simulink model "Demo_PreScanCarSim3D_cs"  (Simulink 7.6)
settings: Solver=ode5  SolverMode=SingleTasking  StartTime=0.0  StopTime=68  FixedStep=1/400  RelTol=1e-3
PreLoadFcn:
  | check_NUTS_defined;
  | 
  | assignin('base',['model_closed_' bdroot],false);
InitFcn:
  | PreScanExperimentInitFcn(bdroot)
StopFcn:
  | PreScanExperimentStopFcn(bdroot)
undefined symbols (not defined in the file or in its folder): DiscIntNeverNeededParam, warningInitialVelocity, x0, x_ini_VRML, y_ini_VRML, z_ini_VRML
libraries: PreScanSimulinkLibrary x13, simulink_extras x5, PreScanUsefulBlocks x5, simulink x3, Solver_SF x1
(part 6 of 10)

== system Demo_PreScanCarSim3D_cs/VISUCasingLights_TrafficLightRoadSideNL_2/conv_Green ==
  on_off : Inport
  Constant5 : Constant  Value=[5 32 25 255 0 64 50 255 0 64 50 255 0 0 0 255]
  Constant9 : Constant  Value="[0 45 34 255  0 45 34 255  0 45 34 255  30 306 240 255]"
  Switch2 : Switch  Threshold=0.5
  RGBcolor : Outport
  wires:
  Switch2/1 -> RGBcolor/1
  on_off/1 -> Switch2/2
  Constant5/1 -> Switch2/3  "off"
  Constant9/1 -> Switch2/1  "on"

== system Demo_PreScanCarSim3D_cs/VISUCasingLights_TrafficLightRoadSideNL_2/conv_Orange ==
  on_off : Inport
  Constant2 : Constant  Value="[45 34 0 255  45 34 0 255  45 34 0 255  306 229 5 255]"
  Constant20 : Constant  Value=[32 25 5 255 64 48 5 255 64 54 5 255 0 0 0 255]
  Switch1 : Switch  Threshold=0.5
  RGBcolor : Outport
  wires:
  Constant20/1 -> Switch1/3  "off"
  Constant2/1 -> Switch1/1  "on"
  on_off/1 -> Switch1/2
  Switch1/1 -> RGBcolor/1

== system Demo_PreScanCarSim3D_cs/VISUCasingLights_TrafficLightRoadSideNL_2/conv_Red ==
  on_off : Inport
  Constant2 : Constant  Value="[45 0 0 255  45 0 0 255  45 0 0 255 306 30 30 255]"
  Constant20 : Constant  Value=[32 5 5 255 64 5 5 255 64 5 5 255 0 0 0 255]
  Switch1 : Switch  Threshold=0.5
  RGBcolor : Outport
  wires:
  Constant20/1 -> Switch1/3  "off"
  Constant2/1 -> Switch1/1  "on"
  on_off/1 -> Switch1/2
  Switch1/1 -> RGBcolor/1

== system Demo_PreScanCarSim3D_cs/VISUCasingLights_TrafficLightRoadSideNL_2/visu_CasingGreen ==
  Y : Inport
  Assignment : Assignment  IndexMode=Zero-based  SampleTime=TimeStep  IndexOptions=Starting index (dialog)  Indices=PortIndex  OutputSizes=[1 1]
  Data Store Read : DataStoreRead  DataStoreName=SimCoreActuators  SampleTime=TimeStep
  Data Store Write : DataStoreWrite  DataStoreName=SimCoreActuators
  wires:
  Assignment/1 -> Data Store Write/1
  Data Store Read/1 -> Assignment/1
  Y/1 -> Assignment/2

== system Demo_PreScanCarSim3D_cs/VISUCasingLights_TrafficLightRoadSideNL_2/visu_CasingOrange ==
  Y : Inport
  Assignment : Assignment  IndexMode=Zero-based  SampleTime=TimeStep  IndexOptions=Starting index (dialog)  Indices=PortIndex  OutputSizes=[1 1]
  Data Store Read : DataStoreRead  DataStoreName=SimCoreActuators  SampleTime=TimeStep
  Data Store Write : DataStoreWrite  DataStoreName=SimCoreActuators
  wires:
  Assignment/1 -> Data Store Write/1
  Data Store Read/1 -> Assignment/1
  Y/1 -> Assignment/2

== system Demo_PreScanCarSim3D_cs/VISUCasingLights_TrafficLightRoadSideNL_2/visu_CasingRed ==
  Y : Inport
  Assignment : Assignment  IndexMode=Zero-based  SampleTime=TimeStep  IndexOptions=Starting index (dialog)  Indices=PortIndex  OutputSizes=[1 1]
  Data Store Read : DataStoreRead  DataStoreName=SimCoreActuators  SampleTime=TimeStep
  Data Store Write : DataStoreWrite  DataStoreName=SimCoreActuators
  wires:
  Assignment/1 -> Data Store Write/1
  Data Store Read/1 -> Assignment/1
  Y/1 -> Assignment/2

== system Demo_PreScanCarSim3D_cs/VISUCasingLights_TrafficLightRoadSideNL_3/conv_Green ==
  on_off : Inport
  Constant5 : Constant  Value=[5 32 25 255 0 64 50 255 0 64 50 255 0 0 0 255]
  Constant9 : Constant  Value="[0 45 34 255  0 45 34 255  0 45 34 255  30 306 240 255]"
  Switch2 : Switch  Threshold=0.5
  RGBcolor : Outport
  wires:
  Switch2/1 -> RGBcolor/1
  on_off/1 -> Switch2/2
  Constant5/1 -> Switch2/3  "off"
  Constant9/1 -> Switch2/1  "on"

== system Demo_PreScanCarSim3D_cs/VISUCasingLights_TrafficLightRoadSideNL_3/conv_Orange ==
  on_off : Inport
  Constant2 : Constant  Value="[45 34 0 255  45 34 0 255  45 34 0 255  306 229 5 255]"
  Constant20 : Constant  Value=[32 25 5 255 64 48 5 255 64 54 5 255 0 0 0 255]
  Switch1 : Switch  Threshold=0.5
  RGBcolor : Outport
  wires:
  Constant20/1 -> Switch1/3  "off"
  Constant2/1 -> Switch1/1  "on"
  on_off/1 -> Switch1/2
  Switch1/1 -> RGBcolor/1

== system Demo_PreScanCarSim3D_cs/VISUCasingLights_TrafficLightRoadSideNL_3/conv_Red ==
  on_off : Inport
  Constant2 : Constant  Value="[45 0 0 255  45 0 0 255  45 0 0 255 306 30 30 255]"
  Constant20 : Constant  Value=[32 5 5 255 64 5 5 255 64 5 5 255 0 0 0 255]
  Switch1 : Switch  Threshold=0.5
  RGBcolor : Outport
  wires:
  Constant20/1 -> Switch1/3  "off"
  Constant2/1 -> Switch1/1  "on"
  on_off/1 -> Switch1/2
  Switch1/1 -> RGBcolor/1

== system Demo_PreScanCarSim3D_cs/VISUCasingLights_TrafficLightRoadSideNL_3/visu_CasingGreen ==
  Y : Inport
  Assignment : Assignment  IndexMode=Zero-based  SampleTime=TimeStep  IndexOptions=Starting index (dialog)  Indices=PortIndex  OutputSizes=[1 1]
  Data Store Read : DataStoreRead  DataStoreName=SimCoreActuators  SampleTime=TimeStep
  Data Store Write : DataStoreWrite  DataStoreName=SimCoreActuators
  wires:
  Assignment/1 -> Data Store Write/1
  Data Store Read/1 -> Assignment/1
  Y/1 -> Assignment/2

== system Demo_PreScanCarSim3D_cs/VISUCasingLights_TrafficLightRoadSideNL_3/visu_CasingOrange ==
  Y : Inport
  Assignment : Assignment  IndexMode=Zero-based  SampleTime=TimeStep  IndexOptions=Starting index (dialog)  Indices=PortIndex  OutputSizes=[1 1]
  Data Store Read : DataStoreRead  DataStoreName=SimCoreActuators  SampleTime=TimeStep
  Data Store Write : DataStoreWrite  DataStoreName=SimCoreActuators
  wires:
  Assignment/1 -> Data Store Write/1
  Data Store Read/1 -> Assignment/1
  Y/1 -> Assignment/2

== system Demo_PreScanCarSim3D_cs/VISUCasingLights_TrafficLightRoadSideNL_3/visu_CasingRed ==
  Y : Inport
  Assignment : Assignment  IndexMode=Zero-based  SampleTime=TimeStep  IndexOptions=Starting index (dialog)  Indices=PortIndex  OutputSizes=[1 1]
  Data Store Read : DataStoreRead  DataStoreName=SimCoreActuators  SampleTime=TimeStep
  Data Store Write : DataStoreWrite  DataStoreName=SimCoreActuators
  wires:
  Assignment/1 -> Data Store Write/1
  Data Store Read/1 -> Assignment/1
  Y/1 -> Assignment/2

== system Demo_PreScanCarSim3D_cs/VISUCasingLights_TrafficLightRoadSideNL_5/conv_Green ==
  on_off : Inport
  Constant5 : Constant  Value=[5 32 25 255 0 64 50 255 0 64 50 255 0 0 0 255]
  Constant9 : Constant  Value="[0 45 34 255  0 45 34 255  0 45 34 255  30 306 240 255]"
  Switch2 : Switch  Threshold=0.5
  RGBcolor : Outport
  wires:
  Switch2/1 -> RGBcolor/1
  on_off/1 -> Switch2/2
  Constant5/1 -> Switch2/3  "off"
  Constant9/1 -> Switch2/1  "on"

== system Demo_PreScanCarSim3D_cs/VISUCasingLights_TrafficLightRoadSideNL_5/conv_Orange ==
  on_off : Inport
  Constant2 : Constant  Value="[45 34 0 255  45 34 0 255  45 34 0 255  306 229 5 255]"
  Constant20 : Constant  Value=[32 25 5 255 64 48 5 255 64 54 5 255 0 0 0 255]
  Switch1 : Switch  Threshold=0.5
  RGBcolor : Outport
  wires:
  Constant20/1 -> Switch1/3  "off"
  Constant2/1 -> Switch1/1  "on"
  on_off/1 -> Switch1/2
  Switch1/1 -> RGBcolor/1

== system Demo_PreScanCarSim3D_cs/VISUCasingLights_TrafficLightRoadSideNL_5/conv_Red ==
  on_off : Inport
  Constant2 : Constant  Value="[45 0 0 255  45 0 0 255  45 0 0 255 306 30 30 255]"
  Constant20 : Constant  Value=[32 5 5 255 64 5 5 255 64 5 5 255 0 0 0 255]
  Switch1 : Switch  Threshold=0.5
  RGBcolor : Outport
  wires:
  Constant20/1 -> Switch1/3  "off"
  Constant2/1 -> Switch1/1  "on"
  on_off/1 -> Switch1/2
  Switch1/1 -> RGBcolor/1

== system Demo_PreScanCarSim3D_cs/VISUCasingLights_TrafficLightRoadSideNL_5/visu_CasingGreen ==
  Y : Inport
  Assignment : Assignment  IndexMode=Zero-based  SampleTime=TimeStep  IndexOptions=Starting index (dialog)  Indices=PortIndex  OutputSizes=[1 1]
  Data Store Read : DataStoreRead  DataStoreName=SimCoreActuators  SampleTime=TimeStep
  Data Store Write : DataStoreWrite  DataStoreName=SimCoreActuators
  wires:
  Assignment/1 -> Data Store Write/1
  Data Store Read/1 -> Assignment/1
  Y/1 -> Assignment/2

== system Demo_PreScanCarSim3D_cs/VISUCasingLights_TrafficLightRoadSideNL_5/visu_CasingOrange ==
  Y : Inport
  Assignment : Assignment  IndexMode=Zero-based  SampleTime=TimeStep  IndexOptions=Starting index (dialog)  Indices=PortIndex  OutputSizes=[1 1]
  Data Store Read : DataStoreRead  DataStoreName=SimCoreActuators  SampleTime=TimeStep
  Data Store Write : DataStoreWrite  DataStoreName=SimCoreActuators
  wires:
  Assignment/1 -> Data Store Write/1
  Data Store Read/1 -> Assignment/1
  Y/1 -> Assignment/2

== system Demo_PreScanCarSim3D_cs/VISUCasingLights_TrafficLightRoadSideNL_5/visu_CasingRed ==
  Y : Inport
  Assignment : Assignment  IndexMode=Zero-based  SampleTime=TimeStep  IndexOptions=Starting index (dialog)  Indices=PortIndex  OutputSizes=[1 1]
  Data Store Read : DataStoreRead  DataStoreName=SimCoreActuators  SampleTime=TimeStep
  Data Store Write : DataStoreWrite  DataStoreName=SimCoreActuators
  wires:
  Assignment/1 -> Data Store Write/1
  Data Store Read/1 -> Assignment/1
  Y/1 -> Assignment/2

== system Demo_PreScanCarSim3D_cs/VISUCasingLights_TrafficLightRoadSideNL_6/conv_Green ==
  on_off : Inport
  Constant5 : Constant  Value=[5 32 25 255 0 64 50 255 0 64 50 255 0 0 0 255]
  Constant9 : Constant  Value="[0 45 34 255  0 45 34 255  0 45 34 255  30 306 240 255]"
  Switch2 : Switch  Threshold=0.5
  RGBcolor : Outport
  wires:
  Switch2/1 -> RGBcolor/1
  on_off/1 -> Switch2/2
  Constant5/1 -> Switch2/3  "off"
  Constant9/1 -> Switch2/1  "on"

== system Demo_PreScanCarSim3D_cs/VISUCasingLights_TrafficLightRoadSideNL_6/conv_Orange ==
  on_off : Inport
  Constant2 : Constant  Value="[45 34 0 255  45 34 0 255  45 34 0 255  306 229 5 255]"
  Constant20 : Constant  Value=[32 25 5 255 64 48 5 255 64 54 5 255 0 0 0 255]
  Switch1 : Switch  Threshold=0.5
  RGBcolor : Outport
  wires:
  Constant20/1 -> Switch1/3  "off"
  Constant2/1 -> Switch1/1  "on"
  on_off/1 -> Switch1/2
  Switch1/1 -> RGBcolor/1

== system Demo_PreScanCarSim3D_cs/VISUCasingLights_TrafficLightRoadSideNL_6/conv_Red ==
  on_off : Inport
  Constant2 : Constant  Value="[45 0 0 255  45 0 0 255  45 0 0 255 306 30 30 255]"
  Constant20 : Constant  Value=[32 5 5 255 64 5 5 255 64 5 5 255 0 0 0 255]
  Switch1 : Switch  Threshold=0.5
  RGBcolor : Outport
  wires:
  Constant20/1 -> Switch1/3  "off"
  Constant2/1 -> Switch1/1  "on"
  on_off/1 -> Switch1/2
  Switch1/1 -> RGBcolor/1

== system Demo_PreScanCarSim3D_cs/VISUCasingLights_TrafficLightRoadSideNL_6/visu_CasingGreen ==
  Y : Inport
  Assignment : Assignment  IndexMode=Zero-based  SampleTime=TimeStep  IndexOptions=Starting index (dialog)  Indices=PortIndex  OutputSizes=[1 1]
  Data Store Read : DataStoreRead  DataStoreName=SimCoreActuators  SampleTime=TimeStep
  Data Store Write : DataStoreWrite  DataStoreName=SimCoreActuators
  wires:
  Assignment/1 -> Data Store Write/1
  Data Store Read/1 -> Assignment/1
  Y/1 -> Assignment/2

== system Demo_PreScanCarSim3D_cs/VISUCasingLights_TrafficLightRoadSideNL_6/visu_CasingOrange ==
  Y : Inport
  Assignment : Assignment  IndexMode=Zero-based  SampleTime=TimeStep  IndexOptions=Starting index (dialog)  Indices=PortIndex  OutputSizes=[1 1]
  Data Store Read : DataStoreRead  DataStoreName=SimCoreActuators  SampleTime=TimeStep
  Data Store Write : DataStoreWrite  DataStoreName=SimCoreActuators
  wires:
  Assignment/1 -> Data Store Write/1
  Data Store Read/1 -> Assignment/1
  Y/1 -> Assignment/2

== system Demo_PreScanCarSim3D_cs/VISUCasingLights_TrafficLightRoadSideNL_6/visu_CasingRed ==
  Y : Inport
  Assignment : Assignment  IndexMode=Zero-based  SampleTime=TimeStep  IndexOptions=Starting index (dialog)  Indices=PortIndex  OutputSizes=[1 1]
  Data Store Read : DataStoreRead  DataStoreName=SimCoreActuators  SampleTime=TimeStep
  Data Store Write : DataStoreWrite  DataStoreName=SimCoreActuators
  wires:
  Assignment/1 -> Data Store Write/1
  Data Store Read/1 -> Assignment/1
  Y/1 -> Assignment/2

== system Demo_PreScanCarSim3D_cs/VISUCasingLights_TrafficLightRoadSideNL_7/conv_Green ==
  on_off : Inport
  Constant5 : Constant  Value=[5 32 25 255 0 64 50 255 0 64 50 255 0 0 0 255]
  Constant9 : Constant  Value="[0 45 34 255  0 45 34 255  0 45 34 255  30 306 240 255]"
  Switch2 : Switch  Threshold=0.5
  RGBcolor : Outport
  wires:
  Switch2/1 -> RGBcolor/1
  on_off/1 -> Switch2/2
  Constant5/1 -> Switch2/3  "off"
  Constant9/1 -> Switch2/1  "on"

== system Demo_PreScanCarSim3D_cs/VISUCasingLights_TrafficLightRoadSideNL_7/conv_Orange ==
  on_off : Inport
  Constant2 : Constant  Value="[45 34 0 255  45 34 0 255  45 34 0 255  306 229 5 255]"
  Constant20 : Constant  Value=[32 25 5 255 64 48 5 255 64 54 5 255 0 0 0 255]
  Switch1 : Switch  Threshold=0.5
  RGBcolor : Outport
  wires:
  Constant20/1 -> Switch1/3  "off"
  Constant2/1 -> Switch1/1  "on"
  on_off/1 -> Switch1/2
  Switch1/1 -> RGBcolor/1

== system Demo_PreScanCarSim3D_cs/VISUCasingLights_TrafficLightRoadSideNL_7/conv_Red ==
  on_off : Inport
  Constant2 : Constant  Value="[45 0 0 255  45 0 0 255  45 0 0 255 306 30 30 255]"
  Constant20 : Constant  Value=[32 5 5 255 64 5 5 255 64 5 5 255 0 0 0 255]
  Switch1 : Switch  Threshold=0.5
  RGBcolor : Outport
  wires:
  Constant20/1 -> Switch1/3  "off"
  Constant2/1 -> Switch1/1  "on"
  on_off/1 -> Switch1/2
  Switch1/1 -> RGBcolor/1

== system Demo_PreScanCarSim3D_cs/VISUCasingLights_TrafficLightRoadSideNL_7/visu_CasingGreen ==
  Y : Inport
  Assignment : Assignment  IndexMode=Zero-based  SampleTime=TimeStep  IndexOptions=Starting index (dialog)  Indices=PortIndex  OutputSizes=[1 1]
  Data Store Read : DataStoreRead  DataStoreName=SimCoreActuators  SampleTime=TimeStep
  Data Store Write : DataStoreWrite  DataStoreName=SimCoreActuators
  wires:
  Assignment/1 -> Data Store Write/1
  Data Store Read/1 -> Assignment/1
  Y/1 -> Assignment/2

== system Demo_PreScanCarSim3D_cs/VISUCasingLights_TrafficLightRoadSideNL_7/visu_CasingOrange ==
  Y : Inport
  Assignment : Assignment  IndexMode=Zero-based  SampleTime=TimeStep  IndexOptions=Starting index (dialog)  Indices=PortIndex  OutputSizes=[1 1]
  Data Store Read : DataStoreRead  DataStoreName=SimCoreActuators  SampleTime=TimeStep
  Data Store Write : DataStoreWrite  DataStoreName=SimCoreActuators
  wires:
  Assignment/1 -> Data Store Write/1
  Data Store Read/1 -> Assignment/1
  Y/1 -> Assignment/2

== system Demo_PreScanCarSim3D_cs/VISUCasingLights_TrafficLightRoadSideNL_7/visu_CasingRed ==
  Y : Inport
  Assignment : Assignment  IndexMode=Zero-based  SampleTime=TimeStep  IndexOptions=Starting index (dialog)  Indices=PortIndex  OutputSizes=[1 1]
  Data Store Read : DataStoreRead  DataStoreName=SimCoreActuators  SampleTime=TimeStep
  Data Store Write : DataStoreWrite  DataStoreName=SimCoreActuators
  wires:
  Assignment/1 -> Data Store Write/1
  Data Store Read/1 -> Assignment/1
  Y/1 -> Assignment/2

== system Demo_PreScanCarSim3D_cs/VISUMatrixSignLights_HighwayOverhang_1/conv_Orange_1 ==
  on_off : Inport
  Constant2 : Constant  Value="[70 45 0 255  70 45 0 255  70 45 0 255  200 150 0 255]"
  Constant20 : Constant  Value=[70 45 0 255 70 45 0 255 70 45 0 255 0 0 0 255]
  Switch1 : Switch  Threshold=0.5
  RGBcolor : Outport
  wires:
  Constant20/1 -> Switch1/3  "off"
  Constant2/1 -> Switch1/1  "on"
  on_off/1 -> Switch1/2
  Switch1/1 -> RGBcolor/1

== system Demo_PreScanCarSim3D_cs/VISUMatrixSignLights_HighwayOverhang_1/conv_Orange_10 ==
  on_off : Inport
  Constant2 : Constant  Value="[70 45 0 255  70 45 0 255  70 45 0 255  200 150 0 255]"
  Constant20 : Constant  Value=[70 45 0 255 70 45 0 255 70 45 0 255 0 0 0 255]
  Switch1 : Switch  Threshold=0.5
  RGBcolor : Outport
  wires:
  Switch1/1 -> RGBcolor/1
  on_off/1 -> Switch1/2
  Constant2/1 -> Switch1/1  "on"
  Constant20/1 -> Switch1/3  "off"

== system Demo_PreScanCarSim3D_cs/VISUMatrixSignLights_HighwayOverhang_1/conv_Orange_11 ==
  on_off : Inport
  Constant2 : Constant  Value="[70 45 0 255  70 45 0 255  70 45 0 255  200 150 0 255]"
  Constant20 : Constant  Value=[70 45 0 255 70 45 0 255 70 45 0 255 0 0 0 255]
  Switch1 : Switch  Threshold=0.5
  RGBcolor : Outport
  wires:
  Switch1/1 -> RGBcolor/1
  on_off/1 -> Switch1/2
  Constant2/1 -> Switch1/1  "on"
  Constant20/1 -> Switch1/3  "off"

== system Demo_PreScanCarSim3D_cs/VISUMatrixSignLights_HighwayOverhang_1/conv_Orange_12 ==
  on_off : Inport
  Constant2 : Constant  Value="[70 45 0 255  70 45 0 255  70 45 0 255  200 150 0 255]"
  Constant20 : Constant  Value=[70 45 0 255 70 45 0 255 70 45 0 255 0 0 0 255]
  Switch1 : Switch  Threshold=0.5
  RGBcolor : Outport
  wires:
  Switch1/1 -> RGBcolor/1
  on_off/1 -> Switch1/2
  Constant2/1 -> Switch1/1  "on"
  Constant20/1 -> Switch1/3  "off"

== system Demo_PreScanCarSim3D_cs/VISUMatrixSignLights_HighwayOverhang_1/conv_Orange_13 ==
  on_off : Inport
  Constant2 : Constant  Value="[70 45 0 255  70 45 0 255  70 45 0 255  200 150 0 255]"
  Constant20 : Constant  Value=[70 45 0 255 70 45 0 255 70 45 0 255 0 0 0 255]
  Switch1 : Switch  Threshold=0.5
  RGBcolor : Outport
  wires:
  Switch1/1 -> RGBcolor/1
  on_off/1 -> Switch1/2
  Constant2/1 -> Switch1/1  "on"
  Constant20/1 -> Switch1/3  "off"

== system Demo_PreScanCarSim3D_cs/VISUMatrixSignLights_HighwayOverhang_1/conv_Orange_14 ==
  on_off : Inport
  Constant2 : Constant  Value="[70 45 0 255  70 45 0 255  70 45 0 255  200 150 0 255]"
  Constant20 : Constant  Value=[70 45 0 255 70 45 0 255 70 45 0 255 0 0 0 255]
  Switch1 : Switch  Threshold=0.5
  RGBcolor : Outport
  wires:
  Switch1/1 -> RGBcolor/1
  on_off/1 -> Switch1/2
  Constant2/1 -> Switch1/1  "on"
  Constant20/1 -> Switch1/3  "off"

== system Demo_PreScanCarSim3D_cs/VISUMatrixSignLights_HighwayOverhang_1/conv_Orange_15 ==
  on_off : Inport
  Constant2 : Constant  Value="[70 45 0 255  70 45 0 255  70 45 0 255  200 150 0 255]"
  Constant20 : Constant  Value=[70 45 0 255 70 45 0 255 70 45 0 255 0 0 0 255]
  Switch1 : Switch  Threshold=0.5
  RGBcolor : Outport
  wires:
  Switch1/1 -> RGBcolor/1
  on_off/1 -> Switch1/2
  Constant2/1 -> Switch1/1  "on"
  Constant20/1 -> Switch1/3  "off"

== system Demo_PreScanCarSim3D_cs/VISUMatrixSignLights_HighwayOverhang_1/conv_Orange_16 ==
  on_off : Inport
  Constant2 : Constant  Value="[70 45 0 255  70 45 0 255  70 45 0 255  200 150 0 255]"
  Constant20 : Constant  Value=[70 45 0 255 70 45 0 255 70 45 0 255 0 0 0 255]
  Switch1 : Switch  Threshold=0.5
  RGBcolor : Outport
  wires:
  Switch1/1 -> RGBcolor/1
  on_off/1 -> Switch1/2
  Constant2/1 -> Switch1/1  "on"
  Constant20/1 -> Switch1/3  "off"

== system Demo_PreScanCarSim3D_cs/VISUMatrixSignLights_HighwayOverhang_1/conv_Orange_2 ==
  on_off : Inport
  Constant2 : Constant  Value="[70 45 0 255  70 45 0 255  70 45 0 255  200 150 0 255]"
  Constant20 : Constant  Value=[70 45 0 255 70 45 0 255 70 45 0 255 0 0 0 255]
  Switch1 : Switch  Threshold=0.5
  RGBcolor : Outport
  wires:
  Switch1/1 -> RGBcolor/1
  on_off/1 -> Switch1/2
  Constant2/1 -> Switch1/1  "on"
  Constant20/1 -> Switch1/3  "off"

== system Demo_PreScanCarSim3D_cs/VISUMatrixSignLights_HighwayOverhang_1/conv_Orange_3 ==
  on_off : Inport
  Constant2 : Constant  Value="[70 45 0 255  70 45 0 255  70 45 0 255  200 150 0 255]"
  Constant20 : Constant  Value=[70 45 0 255 70 45 0 255 70 45 0 255 0 0 0 255]
  Switch1 : Switch  Threshold=0.5
  RGBcolor : Outport
  wires:
  Switch1/1 -> RGBcolor/1
  on_off/1 -> Switch1/2
  Constant2/1 -> Switch1/1  "on"
  Constant20/1 -> Switch1/3  "off"

== system Demo_PreScanCarSim3D_cs/VISUMatrixSignLights_HighwayOverhang_1/conv_Orange_4 ==
  on_off : Inport
  Constant2 : Constant  Value="[70 45 0 255  70 45 0 255  70 45 0 255  200 150 0 255]"
  Constant20 : Constant  Value=[70 45 0 255 70 45 0 255 70 45 0 255 0 0 0 255]
  Switch1 : Switch  Threshold=0.5
  RGBcolor : Outport
  wires:
  Switch1/1 -> RGBcolor/1
  on_off/1 -> Switch1/2
  Constant2/1 -> Switch1/1  "on"
  Constant20/1 -> Switch1/3  "off"

== system Demo_PreScanCarSim3D_cs/VISUMatrixSignLights_HighwayOverhang_1/conv_Orange_5 ==
  on_off : Inport
  Constant2 : Constant  Value="[70 45 0 255  70 45 0 255  70 45 0 255  200 150 0 255]"
  Constant20 : Constant  Value=[70 45 0 255 70 45 0 255 70 45 0 255 0 0 0 255]
  Switch1 : Switch  Threshold=0.5
  RGBcolor : Outport
  wires:
  Switch1/1 -> RGBcolor/1
  on_off/1 -> Switch1/2
  Constant2/1 -> Switch1/1  "on"
  Constant20/1 -> Switch1/3  "off"

== system Demo_PreScanCarSim3D_cs/VISUMatrixSignLights_HighwayOverhang_1/conv_Orange_6 ==
  on_off : Inport
  Constant2 : Constant  Value="[70 45 0 255  70 45 0 255  70 45 0 255  200 150 0 255]"
  Constant20 : Constant  Value=[70 45 0 255 70 45 0 255 70 45 0 255 0 0 0 255]
  Switch1 : Switch  Threshold=0.5
  RGBcolor : Outport
  wires:
  Switch1/1 -> RGBcolor/1
  on_off/1 -> Switch1/2
  Constant2/1 -> Switch1/1  "on"
  Constant20/1 -> Switch1/3  "off"

== system Demo_PreScanCarSim3D_cs/VISUMatrixSignLights_HighwayOverhang_1/conv_Orange_7 ==
  on_off : Inport
  Constant2 : Constant  Value="[70 45 0 255  70 45 0 255  70 45 0 255  200 150 0 255]"
  Constant20 : Constant  Value=[70 45 0 255 70 45 0 255 70 45 0 255 0 0 0 255]
  Switch1 : Switch  Threshold=0.5
  RGBcolor : Outport
  wires:
  Switch1/1 -> RGBcolor/1
  on_off/1 -> Switch1/2
  Constant2/1 -> Switch1/1  "on"
  Constant20/1 -> Switch1/3  "off"

== system Demo_PreScanCarSim3D_cs/VISUMatrixSignLights_HighwayOverhang_1/conv_Orange_8 ==
  on_off : Inport
  Constant2 : Constant  Value="[70 45 0 255  70 45 0 255  70 45 0 255  200 150 0 255]"
  Constant20 : Constant  Value=[70 45 0 255 70 45 0 255 70 45 0 255 0 0 0 255]
  Switch1 : Switch  Threshold=0.5
  RGBcolor : Outport
  wires:
  Switch1/1 -> RGBcolor/1
  on_off/1 -> Switch1/2
  Constant2/1 -> Switch1/1  "on"
  Constant20/1 -> Switch1/3  "off"

== system Demo_PreScanCarSim3D_cs/VISUMatrixSignLights_HighwayOverhang_1/conv_Orange_9 ==
  on_off : Inport
  Constant2 : Constant  Value="[70 45 0 255  70 45 0 255  70 45 0 255  200 150 0 255]"
  Constant20 : Constant  Value=[70 45 0 255 70 45 0 255 70 45 0 255 0 0 0 255]
  Switch1 : Switch  Threshold=0.5
  RGBcolor : Outport
  wires:
  Switch1/1 -> RGBcolor/1
  on_off/1 -> Switch1/2
  Constant2/1 -> Switch1/1  "on"
  Constant20/1 -> Switch1/3  "off"

== system Demo_PreScanCarSim3D_cs/VISUMatrixSignLights_HighwayOverhang_1/visu_MatrixSignLights_1 ==
  Y : Inport
  Assignment : Assignment  IndexMode=Zero-based  SampleTime=TimeStep  IndexOptions=Starting index (dialog)  Indices=PortIndex  OutputSizes=[1 1]
  Data Store Read : DataStoreRead  DataStoreName=SimCoreActuators  SampleTime=TimeStep
  Data Store Write : DataStoreWrite  DataStoreName=SimCoreActuators
  wires:
  Y/1 -> Assignment/2
  Data Store Read/1 -> Assignment/1
  Assignment/1 -> Data Store Write/1

== system Demo_PreScanCarSim3D_cs/VISUMatrixSignLights_HighwayOverhang_1/visu_MatrixSignLights_10 ==
  Y : Inport
  Assignment : Assignment  IndexMode=Zero-based  SampleTime=TimeStep  IndexOptions=Starting index (dialog)  Indices=PortIndex  OutputSizes=[1 1]
  Data Store Read : DataStoreRead  DataStoreName=SimCoreActuators  SampleTime=TimeStep
  Data Store Write : DataStoreWrite  DataStoreName=SimCoreActuators
  wires:
  Assignment/1 -> Data Store Write/1
  Data Store Read/1 -> Assignment/1
  Y/1 -> Assignment/2

== system Demo_PreScanCarSim3D_cs/VISUMatrixSignLights_HighwayOverhang_1/visu_MatrixSignLights_11 ==
  Y : Inport
  Assignment : Assignment  IndexMode=Zero-based  SampleTime=TimeStep  IndexOptions=Starting index (dialog)  Indices=PortIndex  OutputSizes=[1 1]
  Data Store Read : DataStoreRead  DataStoreName=SimCoreActuators  SampleTime=TimeStep
  Data Store Write : DataStoreWrite  DataStoreName=SimCoreActuators
  wires:
  Assignment/1 -> Data Store Write/1
  Data Store Read/1 -> Assignment/1
  Y/1 -> Assignment/2

== system Demo_PreScanCarSim3D_cs/VISUMatrixSignLights_HighwayOverhang_1/visu_MatrixSignLights_12 ==
  Y : Inport
  Assignment : Assignment  IndexMode=Zero-based  SampleTime=TimeStep  IndexOptions=Starting index (dialog)  Indices=PortIndex  OutputSizes=[1 1]
  Data Store Read : DataStoreRead  DataStoreName=SimCoreActuators  SampleTime=TimeStep
  Data Store Write : DataStoreWrite  DataStoreName=SimCoreActuators
  wires:
  Assignment/1 -> Data Store Write/1
  Data Store Read/1 -> Assignment/1
  Y/1 -> Assignment/2

== system Demo_PreScanCarSim3D_cs/VISUMatrixSignLights_HighwayOverhang_1/visu_MatrixSignLights_13 ==
  Y : Inport
  Assignment : Assignment  IndexMode=Zero-based  SampleTime=TimeStep  IndexOptions=Starting index (dialog)  Indices=PortIndex  OutputSizes=[1 1]
  Data Store Read : DataStoreRead  DataStoreName=SimCoreActuators  SampleTime=TimeStep
  Data Store Write : DataStoreWrite  DataStoreName=SimCoreActuators
  wires:
  Assignment/1 -> Data Store Write/1
  Data Store Read/1 -> Assignment/1
  Y/1 -> Assignment/2

== system Demo_PreScanCarSim3D_cs/VISUMatrixSignLights_HighwayOverhang_1/visu_MatrixSignLights_14 ==
  Y : Inport
  Assignment : Assignment  IndexMode=Zero-based  SampleTime=TimeStep  IndexOptions=Starting index (dialog)  Indices=PortIndex  OutputSizes=[1 1]
  Data Store Read : DataStoreRead  DataStoreName=SimCoreActuators  SampleTime=TimeStep
  Data Store Write : DataStoreWrite  DataStoreName=SimCoreActuators
  wires:
  Assignment/1 -> Data Store Write/1
  Data Store Read/1 -> Assignment/1
  Y/1 -> Assignment/2

== system Demo_PreScanCarSim3D_cs/VISUMatrixSignLights_HighwayOverhang_1/visu_MatrixSignLights_15 ==
  Y : Inport
  Assignment : Assignment  IndexMode=Zero-based  SampleTime=TimeStep  IndexOptions=Starting index (dialog)  Indices=PortIndex  OutputSizes=[1 1]
  Data Store Read : DataStoreRead  DataStoreName=SimCoreActuators  SampleTime=TimeStep
  Data Store Write : DataStoreWrite  DataStoreName=SimCoreActuators
  wires:
  Assignment/1 -> Data Store Write/1
  Data Store Read/1 -> Assignment/1
  Y/1 -> Assignment/2

== system Demo_PreScanCarSim3D_cs/VISUMatrixSignLights_HighwayOverhang_1/visu_MatrixSignLights_16 ==
  Y : Inport
  Assignment : Assignment  IndexMode=Zero-based  SampleTime=TimeStep  IndexOptions=Starting index (dialog)  Indices=PortIndex  OutputSizes=[1 1]
  Data Store Read : DataStoreRead  DataStoreName=SimCoreActuators  SampleTime=TimeStep
  Data Store Write : DataStoreWrite  DataStoreName=SimCoreActuators
  wires:
  Assignment/1 -> Data Store Write/1
  Data Store Read/1 -> Assignment/1
  Y/1 -> Assignment/2

== system Demo_PreScanCarSim3D_cs/VISUMatrixSignLights_HighwayOverhang_1/visu_MatrixSignLights_2 ==
  Y : Inport
  Assignment : Assignment  IndexMode=Zero-based  SampleTime=TimeStep  IndexOptions=Starting index (dialog)  Indices=PortIndex  OutputSizes=[1 1]
  Data Store Read : DataStoreRead  DataStoreName=SimCoreActuators  SampleTime=TimeStep
  Data Store Write : DataStoreWrite  DataStoreName=SimCoreActuators
  wires:
  Assignment/1 -> Data Store Write/1
  Data Store Read/1 -> Assignment/1
  Y/1 -> Assignment/2

== system Demo_PreScanCarSim3D_cs/VISUMatrixSignLights_HighwayOverhang_1/visu_MatrixSignLights_3 ==
  Y : Inport
  Assignment : Assignment  IndexMode=Zero-based  SampleTime=TimeStep  IndexOptions=Starting index (dialog)  Indices=PortIndex  OutputSizes=[1 1]
  Data Store Read : DataStoreRead  DataStoreName=SimCoreActuators  SampleTime=TimeStep
  Data Store Write : DataStoreWrite  DataStoreName=SimCoreActuators
  wires:
  Assignment/1 -> Data Store Write/1
  Data Store Read/1 -> Assignment/1
  Y/1 -> Assignment/2

== system Demo_PreScanCarSim3D_cs/VISUMatrixSignLights_HighwayOverhang_1/visu_MatrixSignLights_4 ==
  Y : Inport
  Assignment : Assignment  IndexMode=Zero-based  SampleTime=TimeStep  IndexOptions=Starting index (dialog)  Indices=PortIndex  OutputSizes=[1 1]
  Data Store Read : DataStoreRead  DataStoreName=SimCoreActuators  SampleTime=TimeStep
  Data Store Write : DataStoreWrite  DataStoreName=SimCoreActuators
  wires:
  Assignment/1 -> Data Store Write/1
  Data Store Read/1 -> Assignment/1
  Y/1 -> Assignment/2

== system Demo_PreScanCarSim3D_cs/VISUMatrixSignLights_HighwayOverhang_1/visu_MatrixSignLights_5 ==
  Y : Inport
  Assignment : Assignment  IndexMode=Zero-based  SampleTime=TimeStep  IndexOptions=Starting index (dialog)  Indices=PortIndex  OutputSizes=[1 1]
  Data Store Read : DataStoreRead  DataStoreName=SimCoreActuators  SampleTime=TimeStep
  Data Store Write : DataStoreWrite  DataStoreName=SimCoreActuators
  wires:
  Assignment/1 -> Data Store Write/1
  Data Store Read/1 -> Assignment/1
  Y/1 -> Assignment/2

== system Demo_PreScanCarSim3D_cs/VISUMatrixSignLights_HighwayOverhang_1/visu_MatrixSignLights_6 ==
  Y : Inport
  Assignment : Assignment  IndexMode=Zero-based  SampleTime=TimeStep  IndexOptions=Starting index (dialog)  Indices=PortIndex  OutputSizes=[1 1]
  Data Store Read : DataStoreRead  DataStoreName=SimCoreActuators  SampleTime=TimeStep
  Data Store Write : DataStoreWrite  DataStoreName=SimCoreActuators
  wires:
  Assignment/1 -> Data Store Write/1
  Data Store Read/1 -> Assignment/1
  Y/1 -> Assignment/2

== system Demo_PreScanCarSim3D_cs/VISUMatrixSignLights_HighwayOverhang_1/visu_MatrixSignLights_7 ==
  Y : Inport
  Assignment : Assignment  IndexMode=Zero-based  SampleTime=TimeStep  IndexOptions=Starting index (dialog)  Indices=PortIndex  OutputSizes=[1 1]
  Data Store Read : DataStoreRead  DataStoreName=SimCoreActuators  SampleTime=TimeStep
  Data Store Write : DataStoreWrite  DataStoreName=SimCoreActuators
  wires:
  Assignment/1 -> Data Store Write/1
  Data Store Read/1 -> Assignment/1
  Y/1 -> Assignment/2

== system Demo_PreScanCarSim3D_cs/VISUMatrixSignLights_HighwayOverhang_1/visu_MatrixSignLights_8 ==
  Y : Inport
  Assignment : Assignment  IndexMode=Zero-based  SampleTime=TimeStep  IndexOptions=Starting index (dialog)  Indices=PortIndex  OutputSizes=[1 1]
  Data Store Read : DataStoreRead  DataStoreName=SimCoreActuators  SampleTime=TimeStep
  Data Store Write : DataStoreWrite  DataStoreName=SimCoreActuators
  wires:
  Assignment/1 -> Data Store Write/1
  Data Store Read/1 -> Assignment/1
  Y/1 -> Assignment/2

== system Demo_PreScanCarSim3D_cs/VISUMatrixSignLights_HighwayOverhang_1/visu_MatrixSignLights_9 ==
  Y : Inport
  Assignment : Assignment  IndexMode=Zero-based  SampleTime=TimeStep  IndexOptions=Starting index (dialog)  Indices=PortIndex  OutputSizes=[1 1]
  Data Store Read : DataStoreRead  DataStoreName=SimCoreActuators  SampleTime=TimeStep
  Data Store Write : DataStoreWrite  DataStoreName=SimCoreActuators
  wires:
  Assignment/1 -> Data Store Write/1
  Data Store Read/1 -> Assignment/1
  Y/1 -> Assignment/2

== system Demo_PreScanCarSim3D_cs/VISUMatrixSignLights_HighwayOverhang_2/conv_Orange_1 ==
  on_off : Inport
  Constant2 : Constant  Value="[70 45 0 255  70 45 0 255  70 45 0 255  200 150 0 255]"
  Constant20 : Constant  Value=[70 45 0 255 70 45 0 255 70 45 0 255 0 0 0 255]
  Switch1 : Switch  Threshold=0.5
  RGBcolor : Outport
  wires:
  Constant20/1 -> Switch1/3  "off"
  Constant2/1 -> Switch1/1  "on"
  on_off/1 -> Switch1/2
  Switch1/1 -> RGBcolor/1

== system Demo_PreScanCarSim3D_cs/VISUMatrixSignLights_HighwayOverhang_2/conv_Orange_10 ==
  on_off : Inport
  Constant2 : Constant  Value="[70 45 0 255  70 45 0 255  70 45 0 255  200 150 0 255]"
  Constant20 : Constant  Value=[70 45 0 255 70 45 0 255 70 45 0 255 0 0 0 255]
  Switch1 : Switch  Threshold=0.5
  RGBcolor : Outport
  wires:
  Switch1/1 -> RGBcolor/1
  on_off/1 -> Switch1/2
  Constant2/1 -> Switch1/1  "on"
  Constant20/1 -> Switch1/3  "off"

== system Demo_PreScanCarSim3D_cs/VISUMatrixSignLights_HighwayOverhang_2/conv_Orange_11 ==
  on_off : Inport
  Constant2 : Constant  Value="[70 45 0 255  70 45 0 255  70 45 0 255  200 150 0 255]"
  Constant20 : Constant  Value=[70 45 0 255 70 45 0 255 70 45 0 255 0 0 0 255]
  Switch1 : Switch  Threshold=0.5
  RGBcolor : Outport
  wires:
  Switch1/1 -> RGBcolor/1
  on_off/1 -> Switch1/2
  Constant2/1 -> Switch1/1  "on"
  Constant20/1 -> Switch1/3  "off"

== system Demo_PreScanCarSim3D_cs/VISUMatrixSignLights_HighwayOverhang_2/conv_Orange_12 ==
  on_off : Inport
  Constant2 : Constant  Value="[70 45 0 255  70 45 0 255  70 45 0 255  200 150 0 255]"
  Constant20 : Constant  Value=[70 45 0 255 70 45 0 255 70 45 0 255 0 0 0 255]
  Switch1 : Switch  Threshold=0.5
  RGBcolor : Outport
  wires:
  Switch1/1 -> RGBcolor/1
  on_off/1 -> Switch1/2
  Constant2/1 -> Switch1/1  "on"
  Constant20/1 -> Switch1/3  "off"

== system Demo_PreScanCarSim3D_cs/VISUMatrixSignLights_HighwayOverhang_2/conv_Orange_2 ==
  on_off : Inport
  Constant2 : Constant  Value="[70 45 0 255  70 45 0 255  70 45 0 255  200 150 0 255]"
  Constant20 : Constant  Value=[70 45 0 255 70 45 0 255 70 45 0 255 0 0 0 255]
  Switch1 : Switch  Threshold=0.5
  RGBcolor : Outport
  wires:
  Switch1/1 -> RGBcolor/1
  on_off/1 -> Switch1/2
  Constant2/1 -> Switch1/1  "on"
  Constant20/1 -> Switch1/3  "off"

== system Demo_PreScanCarSim3D_cs/VISUMatrixSignLights_HighwayOverhang_2/conv_Orange_3 ==
  on_off : Inport
  Constant2 : Constant  Value="[70 45 0 255  70 45 0 255  70 45 0 255  200 150 0 255]"
  Constant20 : Constant  Value=[70 45 0 255 70 45 0 255 70 45 0 255 0 0 0 255]
  Switch1 : Switch  Threshold=0.5
  RGBcolor : Outport
  wires:
  Switch1/1 -> RGBcolor/1
  on_off/1 -> Switch1/2
  Constant2/1 -> Switch1/1  "on"
  Constant20/1 -> Switch1/3  "off"

== system Demo_PreScanCarSim3D_cs/VISUMatrixSignLights_HighwayOverhang_2/conv_Orange_4 ==
  on_off : Inport
  Constant2 : Constant  Value="[70 45 0 255  70 45 0 255  70 45 0 255  200 150 0 255]"
  Constant20 : Constant  Value=[70 45 0 255 70 45 0 255 70 45 0 255 0 0 0 255]
  Switch1 : Switch  Threshold=0.5
  RGBcolor : Outport
  wires:
  Switch1/1 -> RGBcolor/1
  on_off/1 -> Switch1/2
  Constant2/1 -> Switch1/1  "on"
  Constant20/1 -> Switch1/3  "off"

== system Demo_PreScanCarSim3D_cs/VISUMatrixSignLights_HighwayOverhang_2/conv_Orange_5 ==
  on_off : Inport
  Constant2 : Constant  Value="[70 45 0 255  70 45 0 255  70 45 0 255  200 150 0 255]"
  Constant20 : Constant  Value=[70 45 0 255 70 45 0 255 70 45 0 255 0 0 0 255]
  Switch1 : Switch  Threshold=0.5
  RGBcolor : Outport
  wires:
  Switch1/1 -> RGBcolor/1
  on_off/1 -> Switch1/2
  Constant2/1 -> Switch1/1  "on"
  Constant20/1 -> Switch1/3  "off"

== system Demo_PreScanCarSim3D_cs/VISUMatrixSignLights_HighwayOverhang_2/conv_Orange_6 ==
  on_off : Inport
  Constant2 : Constant  Value="[70 45 0 255  70 45 0 255  70 45 0 255  200 150 0 255]"
  Constant20 : Constant  Value=[70 45 0 255 70 45 0 255 70 45 0 255 0 0 0 255]
  Switch1 : Switch  Threshold=0.5
  RGBcolor : Outport
  wires:
  Switch1/1 -> RGBcolor/1
  on_off/1 -> Switch1/2
  Constant2/1 -> Switch1/1  "on"
  Constant20/1 -> Switch1/3  "off"

== system Demo_PreScanCarSim3D_cs/VISUMatrixSignLights_HighwayOverhang_2/conv_Orange_7 ==
  on_off : Inport
  Constant2 : Constant  Value="[70 45 0 255  70 45 0 255  70 45 0 255  200 150 0 255]"
  Constant20 : Constant  Value=[70 45 0 255 70 45 0 255 70 45 0 255 0 0 0 255]
  Switch1 : Switch  Threshold=0.5
  RGBcolor : Outport
  wires:
  Switch1/1 -> RGBcolor/1
  on_off/1 -> Switch1/2
  Constant2/1 -> Switch1/1  "on"
  Constant20/1 -> Switch1/3  "off"

== system Demo_PreScanCarSim3D_cs/VISUMatrixSignLights_HighwayOverhang_2/conv_Orange_8 ==
  on_off : Inport
  Constant2 : Constant  Value="[70 45 0 255  70 45 0 255  70 45 0 255  200 150 0 255]"
  Constant20 : Constant  Value=[70 45 0 255 70 45 0 255 70 45 0 255 0 0 0 255]
  Switch1 : Switch  Threshold=0.5
  RGBcolor : Outport
  wires:
  Switch1/1 -> RGBcolor/1
  on_off/1 -> Switch1/2
  Constant2/1 -> Switch1/1  "on"
  Constant20/1 -> Switch1/3  "off"

== system Demo_PreScanCarSim3D_cs/VISUMatrixSignLights_HighwayOverhang_2/conv_Orange_9 ==
  on_off : Inport
  Constant2 : Constant  Value="[70 45 0 255  70 45 0 255  70 45 0 255  200 150 0 255]"
  Constant20 : Constant  Value=[70 45 0 255 70 45 0 255 70 45 0 255 0 0 0 255]
  Switch1 : Switch  Threshold=0.5
  RGBcolor : Outport
  wires:
  Switch1/1 -> RGBcolor/1
  on_off/1 -> Switch1/2
  Constant2/1 -> Switch1/1  "on"
  Constant20/1 -> Switch1/3  "off"

== system Demo_PreScanCarSim3D_cs/VISUMatrixSignLights_HighwayOverhang_2/visu_MatrixSignLights_1 ==
  Y : Inport
  Assignment : Assignment  IndexMode=Zero-based  SampleTime=TimeStep  IndexOptions=Starting index (dialog)  Indices=PortIndex  OutputSizes=[1 1]
  Data Store Read : DataStoreRead  DataStoreName=SimCoreActuators  SampleTime=TimeStep
  Data Store Write : DataStoreWrite  DataStoreName=SimCoreActuators
  wires:
  Y/1 -> Assignment/2
  Data Store Read/1 -> Assignment/1
  Assignment/1 -> Data Store Write/1

== system Demo_PreScanCarSim3D_cs/VISUMatrixSignLights_HighwayOverhang_2/visu_MatrixSignLights_10 ==
  Y : Inport
  Assignment : Assignment  IndexMode=Zero-based  SampleTime=TimeStep  IndexOptions=Starting index (dialog)  Indices=PortIndex  OutputSizes=[1 1]
  Data Store Read : DataStoreRead  DataStoreName=SimCoreActuators  SampleTime=TimeStep
  Data Store Write : DataStoreWrite  DataStoreName=SimCoreActuators
  wires:
  Assignment/1 -> Data Store Write/1
  Data Store Read/1 -> Assignment/1
  Y/1 -> Assignment/2

== system Demo_PreScanCarSim3D_cs/VISUMatrixSignLights_HighwayOverhang_2/visu_MatrixSignLights_11 ==
  Y : Inport
  Assignment : Assignment  IndexMode=Zero-based  SampleTime=TimeStep  IndexOptions=Starting index (dialog)  Indices=PortIndex  OutputSizes=[1 1]
  Data Store Read : DataStoreRead  DataStoreName=SimCoreActuators  SampleTime=TimeStep
  Data Store Write : DataStoreWrite  DataStoreName=SimCoreActuators
  wires:
  Assignment/1 -> Data Store Write/1
  Data Store Read/1 -> Assignment/1
  Y/1 -> Assignment/2

== system Demo_PreScanCarSim3D_cs/VISUMatrixSignLights_HighwayOverhang_2/visu_MatrixSignLights_12 ==
  Y : Inport
  Assignment : Assignment  IndexMode=Zero-based  SampleTime=TimeStep  IndexOptions=Starting index (dialog)  Indices=PortIndex  OutputSizes=[1 1]
  Data Store Read : DataStoreRead  DataStoreName=SimCoreActuators  SampleTime=TimeStep
  Data Store Write : DataStoreWrite  DataStoreName=SimCoreActuators
  wires:
  Assignment/1 -> Data Store Write/1
  Data Store Read/1 -> Assignment/1
  Y/1 -> Assignment/2

== system Demo_PreScanCarSim3D_cs/VISUMatrixSignLights_HighwayOverhang_2/visu_MatrixSignLights_2 ==
  Y : Inport
  Assignment : Assignment  IndexMode=Zero-based  SampleTime=TimeStep  IndexOptions=Starting index (dialog)  Indices=PortIndex  OutputSizes=[1 1]
  Data Store Read : DataStoreRead  DataStoreName=SimCoreActuators  SampleTime=TimeStep
  Data Store Write : DataStoreWrite  DataStoreName=SimCoreActuators
  wires:
  Assignment/1 -> Data Store Write/1
  Data Store Read/1 -> Assignment/1
  Y/1 -> Assignment/2

== system Demo_PreScanCarSim3D_cs/VISUMatrixSignLights_HighwayOverhang_2/visu_MatrixSignLights_3 ==
  Y : Inport
  Assignment : Assignment  IndexMode=Zero-based  SampleTime=TimeStep  IndexOptions=Starting index (dialog)  Indices=PortIndex  OutputSizes=[1 1]
  Data Store Read : DataStoreRead  DataStoreName=SimCoreActuators  SampleTime=TimeStep
  Data Store Write : DataStoreWrite  DataStoreName=SimCoreActuators
  wires:
  Assignment/1 -> Data Store Write/1
  Data Store Read/1 -> Assignment/1
  Y/1 -> Assignment/2

== system Demo_PreScanCarSim3D_cs/VISUMatrixSignLights_HighwayOverhang_2/visu_MatrixSignLights_4 ==
  Y : Inport
  Assignment : Assignment  IndexMode=Zero-based  SampleTime=TimeStep  IndexOptions=Starting index (dialog)  Indices=PortIndex  OutputSizes=[1 1]
  Data Store Read : DataStoreRead  DataStoreName=SimCoreActuators  SampleTime=TimeStep
  Data Store Write : DataStoreWrite  DataStoreName=SimCoreActuators
  wires:
  Assignment/1 -> Data Store Write/1
  Data Store Read/1 -> Assignment/1
  Y/1 -> Assignment/2

== system Demo_PreScanCarSim3D_cs/VISUMatrixSignLights_HighwayOverhang_2/visu_MatrixSignLights_5 ==
  Y : Inport
  Assignment : Assignment  IndexMode=Zero-based  SampleTime=TimeStep  IndexOptions=Starting index (dialog)  Indices=PortIndex  OutputSizes=[1 1]
  Data Store Read : DataStoreRead  DataStoreName=SimCoreActuators  SampleTime=TimeStep
  Data Store Write : DataStoreWrite  DataStoreName=SimCoreActuators
  wires:
  Assignment/1 -> Data Store Write/1
  Data Store Read/1 -> Assignment/1
  Y/1 -> Assignment/2

== system Demo_PreScanCarSim3D_cs/VISUMatrixSignLights_HighwayOverhang_2/visu_MatrixSignLights_6 ==
  Y : Inport
  Assignment : Assignment  IndexMode=Zero-based  SampleTime=TimeStep  IndexOptions=Starting index (dialog)  Indices=PortIndex  OutputSizes=[1 1]
  Data Store Read : DataStoreRead  DataStoreName=SimCoreActuators  SampleTime=TimeStep
  Data Store Write : DataStoreWrite  DataStoreName=SimCoreActuators
  wires:
  Assignment/1 -> Data Store Write/1
  Data Store Read/1 -> Assignment/1
  Y/1 -> Assignment/2

== system Demo_PreScanCarSim3D_cs/VISUMatrixSignLights_HighwayOverhang_2/visu_MatrixSignLights_7 ==
  Y : Inport
  Assignment : Assignment  IndexMode=Zero-based  SampleTime=TimeStep  IndexOptions=Starting index (dialog)  Indices=PortIndex  OutputSizes=[1 1]
  Data Store Read : DataStoreRead  DataStoreName=SimCoreActuators  SampleTime=TimeStep
  Data Store Write : DataStoreWrite  DataStoreName=SimCoreActuators
  wires:
  Assignment/1 -> Data Store Write/1
  Data Store Read/1 -> Assignment/1
  Y/1 -> Assignment/2

== system Demo_PreScanCarSim3D_cs/VISUMatrixSignLights_HighwayOverhang_2/visu_MatrixSignLights_8 ==
  Y : Inport
  Assignment : Assignment  IndexMode=Zero-based  SampleTime=TimeStep  IndexOptions=Starting index (dialog)  Indices=PortIndex  OutputSizes=[1 1]
  Data Store Read : DataStoreRead  DataStoreName=SimCoreActuators  SampleTime=TimeStep
  Data Store Write : DataStoreWrite  DataStoreName=SimCoreActuators
  wires:
  Assignment/1 -> Data Store Write/1
  Data Store Read/1 -> Assignment/1
  Y/1 -> Assignment/2

== system Demo_PreScanCarSim3D_cs/VISUMatrixSignLights_HighwayOverhang_2/visu_MatrixSignLights_9 ==
  Y : Inport
  Assignment : Assignment  IndexMode=Zero-based  SampleTime=TimeStep  IndexOptions=Starting index (dialog)  Indices=PortIndex  OutputSizes=[1 1]
  Data Store Read : DataStoreRead  DataStoreName=SimCoreActuators  SampleTime=TimeStep
  Data Store Write : DataStoreWrite  DataStoreName=SimCoreActuators
  wires:
  Assignment/1 -> Data Store Write/1
  Data Store Read/1 -> Assignment/1
  Y/1 -> Assignment/2

== system Demo_PreScanCarSim3D_cs/VISUMatrixSignLights_HighwayOverhang_3/conv_Orange_1 ==
  on_off : Inport
  Constant2 : Constant  Value="[70 45 0 255  70 45 0 255  70 45 0 255  200 150 0 255]"
  Constant20 : Constant  Value=[70 45 0 255 70 45 0 255 70 45 0 255 0 0 0 255]
  Switch1 : Switch  Threshold=0.5
  RGBcolor : Outport
  wires:
  Constant20/1 -> Switch1/3  "off"
  Constant2/1 -> Switch1/1  "on"
  on_off/1 -> Switch1/2
  Switch1/1 -> RGBcolor/1

== system Demo_PreScanCarSim3D_cs/VISUMatrixSignLights_HighwayOverhang_3/conv_Orange_10 ==
  on_off : Inport
  Constant2 : Constant  Value="[70 45 0 255  70 45 0 255  70 45 0 255  200 150 0 255]"
  Constant20 : Constant  Value=[70 45 0 255 70 45 0 255 70 45 0 255 0 0 0 255]
  Switch1 : Switch  Threshold=0.5
  RGBcolor : Outport
  wires:
  Switch1/1 -> RGBcolor/1
  on_off/1 -> Switch1/2
  Constant2/1 -> Switch1/1  "on"
  Constant20/1 -> Switch1/3  "off"

== system Demo_PreScanCarSim3D_cs/VISUMatrixSignLights_HighwayOverhang_3/conv_Orange_11 ==
  on_off : Inport
  Constant2 : Constant  Value="[70 45 0 255  70 45 0 255  70 45 0 255  200 150 0 255]"
  Constant20 : Constant  Value=[70 45 0 255 70 45 0 255 70 45 0 255 0 0 0 255]
  Switch1 : Switch  Threshold=0.5
  RGBcolor : Outport
  wires:
  Switch1/1 -> RGBcolor/1
  on_off/1 -> Switch1/2
  Constant2/1 -> Switch1/1  "on"
  Constant20/1 -> Switch1/3  "off"

== system Demo_PreScanCarSim3D_cs/VISUMatrixSignLights_HighwayOverhang_3/conv_Orange_12 ==
  on_off : Inport
  Constant2 : Constant  Value="[70 45 0 255  70 45 0 255  70 45 0 255  200 150 0 255]"
  Constant20 : Constant  Value=[70 45 0 255 70 45 0 255 70 45 0 255 0 0 0 255]
  Switch1 : Switch  Threshold=0.5
  RGBcolor : Outport
  wires:
  Switch1/1 -> RGBcolor/1
  on_off/1 -> Switch1/2
  Constant2/1 -> Switch1/1  "on"
  Constant20/1 -> Switch1/3  "off"

== system Demo_PreScanCarSim3D_cs/VISUMatrixSignLights_HighwayOverhang_3/conv_Orange_2 ==
  on_off : Inport
  Constant2 : Constant  Value="[70 45 0 255  70 45 0 255  70 45 0 255  200 150 0 255]"
  Constant20 : Constant  Value=[70 45 0 255 70 45 0 255 70 45 0 255 0 0 0 255]
  Switch1 : Switch  Threshold=0.5
  RGBcolor : Outport
  wires:
  Switch1/1 -> RGBcolor/1
  on_off/1 -> Switch1/2
  Constant2/1 -> Switch1/1  "on"
  Constant20/1 -> Switch1/3  "off"

== system Demo_PreScanCarSim3D_cs/VISUMatrixSignLights_HighwayOverhang_3/conv_Orange_3 ==
  on_off : Inport
  Constant2 : Constant  Value="[70 45 0 255  70 45 0 255  70 45 0 255  200 150 0 255]"
  Constant20 : Constant  Value=[70 45 0 255 70 45 0 255 70 45 0 255 0 0 0 255]
  Switch1 : Switch  Threshold=0.5
  RGBcolor : Outport
  wires:
  Switch1/1 -> RGBcolor/1
  on_off/1 -> Switch1/2
  Constant2/1 -> Switch1/1  "on"
  Constant20/1 -> Switch1/3  "off"

== system Demo_PreScanCarSim3D_cs/VISUMatrixSignLights_HighwayOverhang_3/conv_Orange_4 ==
  on_off : Inport
  Constant2 : Constant  Value="[70 45 0 255  70 45 0 255  70 45 0 255  200 150 0 255]"
  Constant20 : Constant  Value=[70 45 0 255 70 45 0 255 70 45 0 255 0 0 0 255]
  Switch1 : Switch  Threshold=0.5
  RGBcolor : Outport
  wires:
  Switch1/1 -> RGBcolor/1
  on_off/1 -> Switch1/2
  Constant2/1 -> Switch1/1  "on"
  Constant20/1 -> Switch1/3  "off"

== system Demo_PreScanCarSim3D_cs/VISUMatrixSignLights_HighwayOverhang_3/conv_Orange_5 ==
  on_off : Inport
  Constant2 : Constant  Value="[70 45 0 255  70 45 0 255  70 45 0 255  200 150 0 255]"
  Constant20 : Constant  Value=[70 45 0 255 70 45 0 255 70 45 0 255 0 0 0 255]
  Switch1 : Switch  Threshold=0.5
  RGBcolor : Outport
  wires:
  Switch1/1 -> RGBcolor/1
  on_off/1 -> Switch1/2
  Constant2/1 -> Switch1/1  "on"
  Constant20/1 -> Switch1/3  "off"

== system Demo_PreScanCarSim3D_cs/VISUMatrixSignLights_HighwayOverhang_3/conv_Orange_6 ==
  on_off : Inport
  Constant2 : Constant  Value="[70 45 0 255  70 45 0 255  70 45 0 255  200 150 0 255]"
  Constant20 : Constant  Value=[70 45 0 255 70 45 0 255 70 45 0 255 0 0 0 255]
  Switch1 : Switch  Threshold=0.5
  RGBcolor : Outport
  wires:
  Switch1/1 -> RGBcolor/1
  on_off/1 -> Switch1/2
  Constant2/1 -> Switch1/1  "on"
  Constant20/1 -> Switch1/3  "off"

== system Demo_PreScanCarSim3D_cs/VISUMatrixSignLights_HighwayOverhang_3/conv_Orange_7 ==
  on_off : Inport
  Constant2 : Constant  Value="[70 45 0 255  70 45 0 255  70 45 0 255  200 150 0 255]"
  Constant20 : Constant  Value=[70 45 0 255 70 45 0 255 70 45 0 255 0 0 0 255]
  Switch1 : Switch  Threshold=0.5
  RGBcolor : Outport
  wires:
  Switch1/1 -> RGBcolor/1
  on_off/1 -> Switch1/2
  Constant2/1 -> Switch1/1  "on"
  Constant20/1 -> Switch1/3  "off"

== system Demo_PreScanCarSim3D_cs/VISUMatrixSignLights_HighwayOverhang_3/conv_Orange_8 ==
  on_off : Inport
  Constant2 : Constant  Value="[70 45 0 255  70 45 0 255  70 45 0 255  200 150 0 255]"
  Constant20 : Constant  Value=[70 45 0 255 70 45 0 255 70 45 0 255 0 0 0 255]
  Switch1 : Switch  Threshold=0.5
  RGBcolor : Outport
  wires:
  Switch1/1 -> RGBcolor/1
  on_off/1 -> Switch1/2
  Constant2/1 -> Switch1/1  "on"
  Constant20/1 -> Switch1/3  "off"

== system Demo_PreScanCarSim3D_cs/VISUMatrixSignLights_HighwayOverhang_3/conv_Orange_9 ==
  on_off : Inport
  Constant2 : Constant  Value="[70 45 0 255  70 45 0 255  70 45 0 255  200 150 0 255]"
  Constant20 : Constant  Value=[70 45 0 255 70 45 0 255 70 45 0 255 0 0 0 255]
  Switch1 : Switch  Threshold=0.5
  RGBcolor : Outport
  wires:
  Switch1/1 -> RGBcolor/1
  on_off/1 -> Switch1/2
  Constant2/1 -> Switch1/1  "on"
  Constant20/1 -> Switch1/3  "off"

== system Demo_PreScanCarSim3D_cs/VISUMatrixSignLights_HighwayOverhang_3/visu_MatrixSignLights_1 ==
  Y : Inport
  Assignment : Assignment  IndexMode=Zero-based  SampleTime=TimeStep  IndexOptions=Starting index (dialog)  Indices=PortIndex  OutputSizes=[1 1]
  Data Store Read : DataStoreRead  DataStoreName=SimCoreActuators  SampleTime=TimeStep
  Data Store Write : DataStoreWrite  DataStoreName=SimCoreActuators
  wires:
  Y/1 -> Assignment/2
  Data Store Read/1 -> Assignment/1
  Assignment/1 -> Data Store Write/1
